simulink model "comparacion"  (R2021a)
settings: Solver=VariableStepAuto  StartTime=0.0  StopTime=T_fin  RelTol=1e-3
values from neighbouring files (symbols this model uses):
  x0 = [pos(1), 0]    [comparacion_de_modelos.m]    (also in discretizacion.m = [0;0]; obtencion_b.m = x_med(1))
settings Model: Creator=Santiago  LastModifiedBy=Santiago

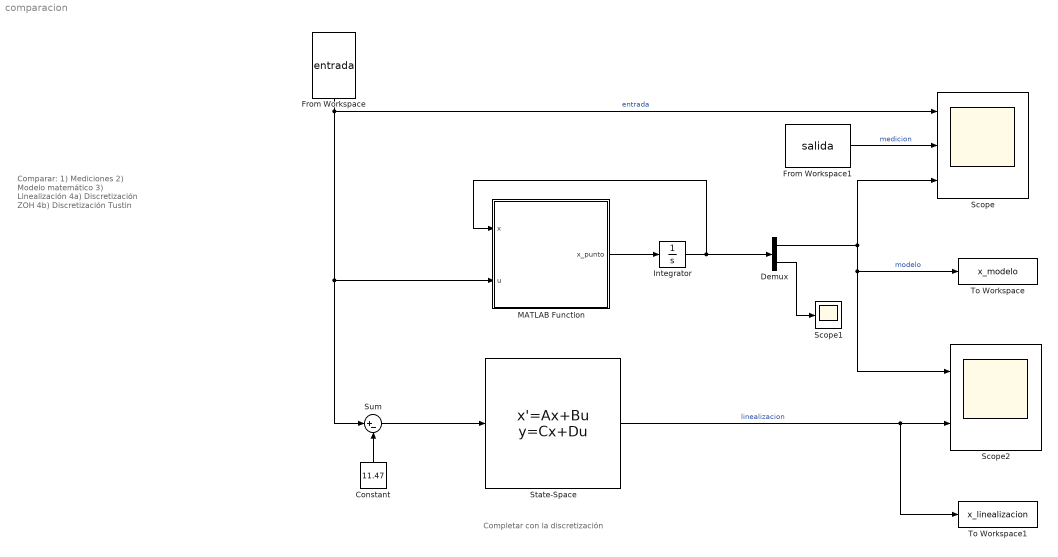
== system comparacion ==
  note: Completar con la discretización
  note: Comparar: 1) Mediciones
      | 2) Modelo matemático
      | 3) Linealización
      | 4a) Discretización ZOH
      | 4b) Discretización Tustin
  Constant : Constant  Value=11.47
  Demux : Demux  Outputs=2
  From Workspace : FromWorkspace  VariableName=entrada
  From Workspace1 : FromWorkspace  VariableName=salida
  Integrator : Integrator  InitialCondition=x0
  MATLAB Function : MATLAB Function  TreatAsAtomicUnit=on
  Scope : Scope  NumInputPorts=3
  Scope1 : Scope
  Scope2 : Scope  NumInputPorts=2
  State-Space : StateSpace  A=[0, 1; 0, -0.15/(33/1000)]  B=[0; 0.34 * 9.8]  C=[1, 0]  D=0  InitialCondition=x0  ParameterTunability=Unconstrained
  Sum : Sum  Inputs=|+-
  To Workspace : ToWorkspace  VariableName=x_modelo  SampleTime=0.02
  To Workspace1 : ToWorkspace  VariableName=x_linealizacion  SampleTime=0.02
  wires:
  MATLAB Function/1(x_punto) -> Integrator/1
  Integrator/1 -> Demux/1, MATLAB Function/1(x)
  From Workspace/1 -> Sum/1, MATLAB Function/2(u), Scope/1  "entrada"
  Demux/2 -> Scope1/1
  Sum/1 -> State-Space/1
  Constant/1 -> Sum/2
  From Workspace1/1 -> Scope/2  "medicion"
  Demux/1 -> To Workspace/1, Scope2/1, Scope/3  "modelo"
  State-Space/1 -> To Workspace1/1, Scope2/2  "linealizacion"

== matlab function comparacion/MATLAB Function ==
  data: x input; u input; x_punto output
function x_punto = fcn(x, u)

b = 0.25; %CORREGIR
g = 9.81;
m = 33/1000; 
a0 = -3.9; %[°]
a1 = 0.34;
x_punto = zeros(2,1);

x_punto(1) = x(2);

theta_b = a0 + a1 * u; %[°]
x_punto(2) = 100 * g * sin(deg2rad(theta_b)) - (b/m)*x(2); %multiplico por 100 para pasar a cm/s^2
end
